simulink model "PID_Controller_final"  (R2014b)
settings: Solver=ode45  StartTime=0.0  StopTime=20  RelTol=1e-3
undefined symbols (not defined in the file or in its folder): sigbuilder_block
libraries: simulink x3
settings Model: Creator=Asus  LastModifiedBy=Asus

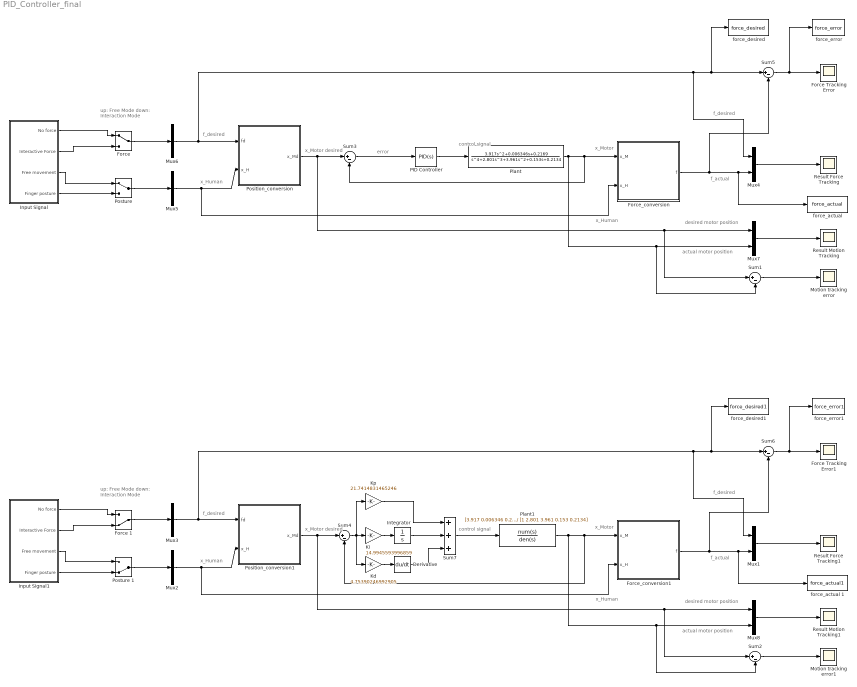
== system PID_Controller_final ==
  note: up:     Free Mode
      | down: Interaction Mode
  note: control signal
  note: error
  note: x_Motor
  note: x_Motor desired
  note: x_Human
  note: actual motor position
  note: desired motor position
  note: f_desired
  note: f_actual
  note: x_Human
  note: f_desired
  note: up:     Free Mode
      | down: Interaction Mode
  note: control signal
  note: x_Motor
  note: x_Motor desired
  note: x_Human
  note: actual motor position
  note: desired motor position
  note: f_desired
  note: f_actual
  note: x_Human
  note: f_desired
  Derivative : Derivative
  "Force " : ManualSwitch
  Force 1 : ManualSwitch  CurrentSetting=0
  Force Tracking Error : Scope
      settings: ShowLegends=on  TimeRange=20  YMin=-5.005624140355663  SaveName=ScopeData5
  Force Tracking Error1 : Scope
      settings: ShowLegends=on  TimeRange=20  YMin=-5.005624140355663
  Force_conversion : MATLAB Function  TreatAsAtomicUnit=on
  Force_conversion1 : MATLAB Function  TreatAsAtomicUnit=on
  Input Signal : Subsystem
  Input Signal1 : Subsystem
  Integrator : Integrator
  Kd : Gain  Gain=4.75390246992905
  Ki : Gain  Gain=14.9945593996859
  Kp : Gain  Gain=21.7414831465246
  Motion tracking error : Scope
      settings: ShowLegends=on
  Motion tracking error1 : Scope
      settings: ShowLegends=on  SaveName=ScopeData2
  Mux{1,4,7..8} (4 alike) : Mux  Inputs=2
  Mux{2..3,5..6} (4 alike) : Mux  Inputs=1
  PID Controller : simulink/Continuous/PID Controller  Controller=PID  TimeDomain=Continuous-time  SampleTime=-1  IntegratorMethod=Forward Euler  FilterMethod=Forward Euler  Form=Parallel  P=21.7414831465246  I=14.9945593996859  D=4.75390246992905  N=106.029452778944  InitialConditionSource=internal  InitialConditionForIntegrator=0  InitialConditionForFilter=0  ExternalReset=none  LimitOutput=off  UpperSaturationLimit=inf  LowerSaturationLimit=-inf  LinearizeAsGain=on  AntiWindupMode=none  Kb=1  TrackingMode=off  Kt=1  PParamMin=[]  PParamMax=[]  IParamMin=[]  IParamMax=[]  DParamMin=[]  DParamMax=[]  NParamMin=[]  NParamMax=[]  KbParamMin=[]  KbParamMax=[]  KtParamMin=[]  KtParamMax=[]  POutMin=[]  POutMax=[]  IOutMin=[]  IOutMax=[]  DOutMin=[]  DOutMax=[]  NOutMin=[]  NOutMax=[]  KbOutMin=[]  KbOutMax=[]  KtOutMin=[]  KtOutMax=[]  IntegratorOutMin=[]  IntegratorOutMax=[]  FilterOutMin=[]  FilterOutMax=[]  SumOutMin=[]  SumOutMax=[]  SumI1OutMin=[]  SumI1OutMax=[]  SumI2OutMin=[]  SumI2OutMax=[]  SumI3OutMin=[]  SumI3OutMax=[]  SumDOutMin=[]  SumDOutMax=[]  SaturationOutMin=[]  SaturationOutMax=[]  IntegratorContinuousStateAttributes=''  IntegratorStateMustResolveToSignalObject=off  IntegratorRTWStateStorageClass=Auto  FilterContinuousStateAttributes=''  FilterStateMustResolveToSignalObject=off  FilterRTWStateStorageClass=Auto  DifferentiatorICPrevScaledInput=0  DifferentiatorOutMin=[]  DifferentiatorOutMax=[]  UseFilter=on
  Plant : TransferFcn  Numerator=[3.917 0.006346 0.2169]  Denominator=[1 2.801 3.961 0.153 0.2134]
  Plant1 : TransferFcn  Numerator=[3.917 0.006346 0.2169]  Denominator=[1 2.801 3.961 0.153 0.2134]
  Position_conversion : MATLAB Function  TreatAsAtomicUnit=on
  Position_conversion1 : MATLAB Function  TreatAsAtomicUnit=on
  "Posture " : ManualSwitch
  Posture 1 : ManualSwitch  CurrentSetting=0
  Result Force Tracking : Scope
      settings: TickLabels=on  ShowLegends=on  SaveName=Result_Force_Tracking
  Result Force Tracking1 : Scope
      settings: TickLabels=on  ShowLegends=on  SaveName=Result_Force_Tracking1
  Result Motion Tracking : Scope
      settings: ShowLegends=on  SaveName=Result_Motion_Tracking
  Result Motion Tracking1 : Scope
      settings: ShowLegends=on  SaveName=Result_Motion_Tracking1
  Sum{1..6} (6 alike) : Sum  Inputs=|+-
  Sum7 : Sum  Inputs=+++
  "force_actual " : ToWorkspace  VariableName=force_actual  SampleTime=-1
      settings: Save2DSignal=2-D array (concatenate along first dimension)
  force_actual 1 : ToWorkspace  VariableName=force_actual1  SampleTime=-1
      settings: Save2DSignal=2-D array (concatenate along first dimension)
  force_desired : ToWorkspace  VariableName=force_desired  SampleTime=-1
      settings: Save2DSignal=2-D array (concatenate along first dimension)
  force_desired1 : ToWorkspace  VariableName=force_desired1  SampleTime=-1
      settings: Save2DSignal=2-D array (concatenate along first dimension)
  force_error : ToWorkspace  VariableName=force_error  SampleTime=-1
      settings: Save2DSignal=2-D array (concatenate along first dimension)
  force_error1 : ToWorkspace  VariableName=force_error1  SampleTime=-1
      settings: Save2DSignal=2-D array (concatenate along first dimension)
  wires:
  Position_conversion/1(x_Md) -> Sum1/1, Mux7/1, Sum3/1
  Force_conversion/1(f) -> Sum5/2, "force_actual "/1, Mux4/2
  Mux5/1 -> Force_conversion/2(x_H), Position_conversion/2(x_H)
  Mux6/1 -> Mux4/1, force_desired/1, Sum5/1, Position_conversion/1(fd)
  Mux7/1 -> Result Motion Tracking/1
  Sum5/1 -> force_error/1, Force Tracking Error/1
  Mux4/1 -> Result Force Tracking/1
  Sum1/1 -> Motion tracking error/1
  Sum3/1 -> PID Controller/1
  PID Controller/1 -> Plant/1
  "Force "/1 -> Mux6/1
  "Posture "/1 -> Mux5/1
  Plant/1 -> Sum1/2, Mux7/2, Sum3/2, Force_conversion/1(x_M)
  Input Signal/1("No force ") -> "Force "/1
  Input Signal/2(Interactive Force) -> "Force "/2
  Input Signal/3(Free movement) -> "Posture "/1
  Input Signal/4(Finger posture) -> "Posture "/2
  Position_conversion1/1(x_Md) -> Sum2/1, Mux8/1, Sum4/1
  Force_conversion1/1(f) -> Sum6/2, force_actual 1/1, Mux1/2
  Mux2/1 -> Force_conversion1/2(x_H), Position_conversion1/2(x_H)
  Mux3/1 -> Mux1/1, force_desired1/1, Sum6/1, Position_conversion1/1(fd)
  Mux8/1 -> Result Motion Tracking1/1
  Sum6/1 -> force_error1/1, Force Tracking Error1/1
  Mux1/1 -> Result Force Tracking1/1
  Sum2/1 -> Motion tracking error1/1
  Force 1/1 -> Mux3/1
  Posture 1/1 -> Mux2/1
  Plant1/1 -> Sum2/2, Mux8/2, Sum4/2, Force_conversion1/1(x_M)
  Input Signal1/1("No force ") -> Force 1/1
  Input Signal1/2(Interactive Force) -> Force 1/2
  Input Signal1/3(Free movement) -> Posture 1/1
  Input Signal1/4(Finger posture) -> Posture 1/2
  Sum7/1 -> Plant1/1
  Kd/1 -> Derivative/1
  Sum4/1 -> Kd/1, Kp/1, Ki/1
  Ki/1 -> Integrator/1
  Kp/1 -> Sum7/1
  Integrator/1 -> Sum7/2
  Derivative/1 -> Sum7/3

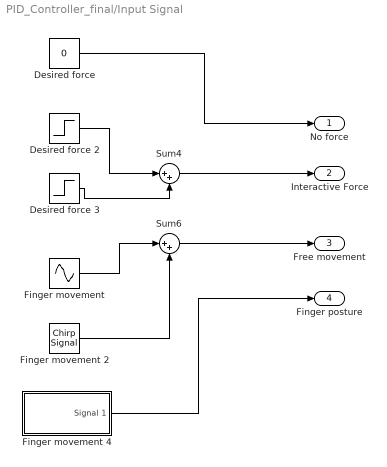
== system PID_Controller_final/Input Signal ==
  Desired force : Constant  Value=0
  Desired force 2 : Step  Time=3  After=5  SampleTime=0
  Desired force 3 : Step  Time=6  After=-5  SampleTime=0
  Finger movement : Sin  Bias=8  Frequency=2  Samples=20  SampleTime=0
  Finger movement 2 : simulink/Sources/Chirp Signal  f1=0  T=20  f2=1
  Finger movement 4 : Subsystem  Tag=STV Subsys  LoadFcn=sigbuilder_block('load');  StartFcn=sigbuilder_block('start');  StopFcn=sigbuilder_block('stop');  ClipboardFcn=sigbuilder_block('clipboard');  mask(Sigbuilder block){}
      mask help: Simulink:masks:SigbuilderBlock_MD
      mask init:
      | if ~strcmp(get_param(bdroot(gcbh),'SimulationStatus'),'stopped') tuvar = sigbuilder_block('maskInit'); end
      settings: CopyFcn=sigbuilder_block('copy');  DeleteFcn=sigbuilder_block('delete');  ModelCloseFcn=sigbuilder_block('modelClose');  PreSaveFcn=sigbuilder_block('preSave');  PauseFcn=sigbuilder_block('pause');  ContinueFcn=sigbuilder_block('continue');  NameChangeFcn=sigbuilder_block('namechange');  OpenFcn=sigbuilder_block('open',[437.6 199.2 550.4 400 ]);  CloseFcn=sigbuilder_block('close');
      mask Display: plot(0, 0, 100, 100,[2, 2, 32, 32, 2], [68, 8, 8, 68, 68],[32, 2], [38, 38], [32, 19, 2],[53, 60, 44], [32, 17, 17, 2],[16, 16, 31, 31]);txt = getActiveGroup(gcbh);text(2, 100, txt,'verticalAlignment', 'top');
  Sum4 : Sum  Inputs=|++
  Sum6 : Sum  Inputs=|++
  "No force " : Outport
  Interactive Force : Outport  Port=2
  Free movement : Outport  Port=3
  Finger posture : Outport  Port=4
  wires:
  Desired force 3/1 -> Sum4/2
  Finger movement/1 -> Sum6/1
  Sum6/1 -> Free movement/1
  Finger movement 2/1 -> Sum6/2
  Finger movement 4/1(Signal 1) -> Finger posture/1
  Desired force/1 -> "No force "/1
  Desired force 2/1 -> Sum4/1
  Sum4/1 -> Interactive Force/1

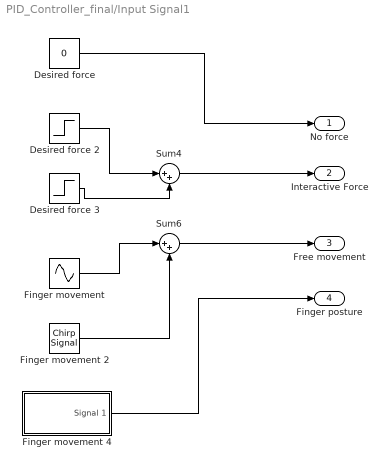
== system PID_Controller_final/Input Signal1 ==
  Desired force : Constant  Value=0
  Desired force 2 : Step  Time=3  After=5  SampleTime=0
  Desired force 3 : Step  Time=6  After=-5  SampleTime=0
  Finger movement : Sin  Bias=8  Frequency=2  Samples=20  SampleTime=0
  Finger movement 2 : simulink/Sources/Chirp Signal  f1=0  T=20  f2=1
  Finger movement 4 : Subsystem  Tag=STV Subsys  LoadFcn=sigbuilder_block('load');  StartFcn=sigbuilder_block('start');  StopFcn=sigbuilder_block('stop');  ClipboardFcn=sigbuilder_block('clipboard');  mask(Sigbuilder block){}
      mask help: Simulink:masks:SigbuilderBlock_MD
      mask init:
      | if ~strcmp(get_param(bdroot(gcbh),'SimulationStatus'),'stopped') tuvar = sigbuilder_block('maskInit'); end
      settings: CopyFcn=sigbuilder_block('copy');  DeleteFcn=sigbuilder_block('delete');  ModelCloseFcn=sigbuilder_block('modelClose');  PreSaveFcn=sigbuilder_block('preSave');  PauseFcn=sigbuilder_block('pause');  ContinueFcn=sigbuilder_block('continue');  NameChangeFcn=sigbuilder_block('namechange');  OpenFcn=sigbuilder_block('open',[437.6 199.2 550.4 400 ]);  CloseFcn=sigbuilder_block('close');
      mask Display: plot(0, 0, 100, 100,[2, 2, 32, 32, 2], [68, 8, 8, 68, 68],[32, 2], [38, 38], [32, 19, 2],[53, 60, 44], [32, 17, 17, 2],[16, 16, 31, 31]);txt = getActiveGroup(gcbh);text(2, 100, txt,'verticalAlignment', 'top');
  Sum4 : Sum  Inputs=|++
  Sum6 : Sum  Inputs=|++
  "No force " : Outport
  Interactive Force : Outport  Port=2
  Free movement : Outport  Port=3
  Finger posture : Outport  Port=4
  wires:
  Desired force 3/1 -> Sum4/2
  Finger movement/1 -> Sum6/1
  Sum6/1 -> Free movement/1
  Finger movement 2/1 -> Sum6/2
  Finger movement 4/1(Signal 1) -> Finger posture/1
  Desired force/1 -> "No force "/1
  Desired force 2/1 -> Sum4/1
  Sum4/1 -> Interactive Force/1

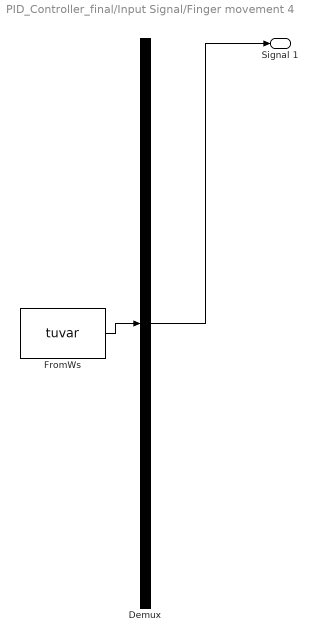
== system PID_Controller_final/Input Signal/Finger movement 4 ==
  Demux : Demux  Tag=STV Demux  Outputs=1
  FromWs : FromWorkspace  Tag=STV FromWs  VariableName=tuvar  SampleTime=0
      SigBuilderData=|
      | common.afterFinalStr = 'Extrapolate'
      | common.sampleTime = 0
      | dataSet.timeRange = [0 10]
      | dataSet.name = 'Group 1'
      | sbobj.Groups.Name = 'Group 1'
      | sbobj.Groups.Signals.Name = 'Signal 1'
      | sbobj.Groups.Signals.XData = [0 3 6 10]
      | sbobj.Groups.Signals.YData = [8 13 13 8]
  Signal 1 : Outport  Tag=STV Outport
  wires:
  Demux/1 -> Signal 1/1
  FromWs/1 -> Demux/1

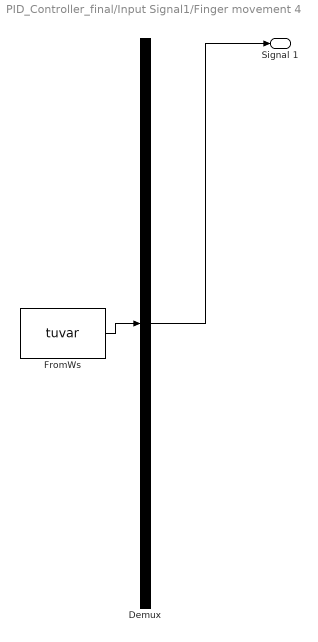
== system PID_Controller_final/Input Signal1/Finger movement 4 ==
  Demux : Demux  Tag=STV Demux  Outputs=1
  FromWs : FromWorkspace  Tag=STV FromWs  VariableName=tuvar  SampleTime=0
      SigBuilderData=|
      | common.afterFinalStr = 'Extrapolate'
      | common.sampleTime = 0
      | dataSet.timeRange = [0 10]
      | dataSet.name = 'Group 1'
      | sbobj.Groups.Name = 'Group 1'
      | sbobj.Groups.Signals.Name = 'Signal 1'
      | sbobj.Groups.Signals.XData = [0 3 6 10]
      | sbobj.Groups.Signals.YData = [8 13 13 8]
  Signal 1 : Outport  Tag=STV Outport
  wires:
  Demux/1 -> Signal 1/1
  FromWs/1 -> Demux/1

== matlab function PID_Controller_final/Force_conversion ==
  data: x_M input; f output; x_H input
function f = force_conver(x_M,x_H)
%#codegen
    k = 0.434;
    L0 = 8;
    f = k*(x_H - x_M - L0);
end

== matlab function PID_Controller_final/Position_conversion ==
  data: fd input; x_Md output; x_H input
function x_Md = pos_conver(fd,x_H)
%#codegen
    k = 0.434; %N/mm
    L0 = 8;    %mm
    x_Md = x_H - (fd/k) - L0;
end

== matlab function PID_Controller_final/Force_conversion1 ==
  data: x_M input; f output; x_H input
function f = force_conver(x_M,x_H)
%#codegen
    k = 0.434;
    L0 = 8;
    f = k*(x_H - x_M - L0);
end

== matlab function PID_Controller_final/Position_conversion1 ==
  data: fd input; x_Md output; x_H input
function x_Md = pos_conver(fd,x_H)
%#codegen
    k = 0.434; %N/mm
    L0 = 8;    %mm
    x_Md = x_H - (fd/k) - L0;
end
